simulink model "PWMGenerator"  (R2018a)
settings: Solver=VariableStepAuto  StartTime=0.0  StopTime=10.0  RelTol=1e-3
libraries: hdlsllib x15, simulink x5
settings Model: Creator=prasad.ra  LastModifiedBy=prasad.ra
settings OptimizationCC: BlockReduction=off  ConditionallyExecuteInputs=off  DefaultParameterBehavior=Inlined
settings DebuggingCC: AlgebraicLoopMsg=error
settings HardwareCC: ProdBitPerPointer=32  ProdBitPerSizeT=32  ProdBitPerPtrDiffT=32  ProdLargestAtomicFloat=None  ProdIntDivRoundTo=Undefined  ProdEndianess=Unspecified  ProdWordSize=32  ProdHWDeviceType=ASIC/FPGA->ASIC/FPGA  TargetBitPerPointer=64  TargetBitPerSizeT=64  TargetBitPerPtrDiffT=64  TargetLongLongMode=on  TargetIntDivRoundTo=Zero  TargetEndianess=LittleEndian  TargetWordSize=64  TargetHWDeviceType=Custom Processor->MATLAB Host Computer  ProdEqTarget=off

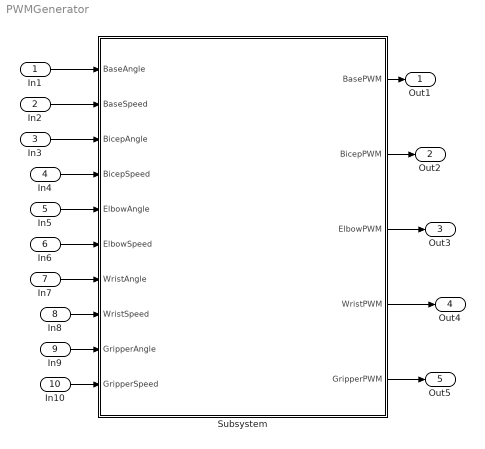
== system PWMGenerator ==
  In1 : Inport
  In2 : Inport  Port=2
  In3 : Inport  Port=3
  In4 : Inport  Port=4
  In5 : Inport  Port=5
  In6 : Inport  Port=6
  In7 : Inport  Port=7
  In8 : Inport  Port=8
  In9 : Inport  Port=9
  In10 : Inport  Port=10
  Subsystem : Subsystem
  Out1 : Outport
  Out2 : Outport  Port=2
  Out3 : Outport  Port=3
  Out4 : Outport  Port=4
  Out5 : Outport  Port=5
  wires:
  In1/1 -> Subsystem/1(BaseAngle)
  In2/1 -> Subsystem/2(BaseSpeed)
  In3/1 -> Subsystem/3(BicepAngle)
  In4/1 -> Subsystem/4(BicepSpeed)
  In7/1 -> Subsystem/7(WristAngle)
  In6/1 -> Subsystem/6(ElbowSpeed)
  In5/1 -> Subsystem/5(ElbowAngle)
  In8/1 -> Subsystem/8(WristSpeed)
  In9/1 -> Subsystem/9(GripperAngle)
  In10/1 -> Subsystem/10(GripperSpeed)
  Subsystem/1(BasePWM) -> Out1/1
  Subsystem/2(BicepPWM) -> Out2/1
  Subsystem/3(ElbowPWM) -> Out3/1
  Subsystem/4(WristPWM) -> Out4/1
  Subsystem/5(GripperPWM) -> Out5/1

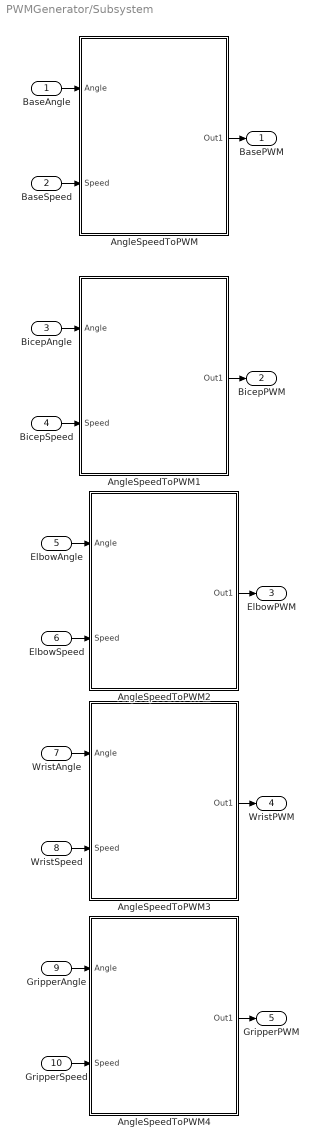
== system PWMGenerator/Subsystem ==
  BaseAngle : Inport
  BaseSpeed : Inport  Port=2
  BicepAngle : Inport  Port=3
  BicepSpeed : Inport  Port=4
  ElbowAngle : Inport  Port=5
  ElbowSpeed : Inport  Port=6
  WristAngle : Inport  Port=7
  WristSpeed : Inport  Port=8
  GripperAngle : Inport  Port=9
  GripperSpeed : Inport  Port=10
  AngleSpeedToPWM : Subsystem
  AngleSpeedToPWM1 : Subsystem
  AngleSpeedToPWM2 : Subsystem
  AngleSpeedToPWM3 : Subsystem
  AngleSpeedToPWM4 : Subsystem
  BasePWM : Outport
  BicepPWM : Outport  Port=2
  ElbowPWM : Outport  Port=3
  WristPWM : Outport  Port=4
  GripperPWM : Outport  Port=5
  wires:
  BicepSpeed/1 -> AngleSpeedToPWM1/2("Speed ")
  AngleSpeedToPWM/1(Out1) -> BasePWM/1
  ElbowSpeed/1 -> AngleSpeedToPWM2/2("Speed ")
  AngleSpeedToPWM2/1(Out1) -> ElbowPWM/1
  BaseAngle/1 -> AngleSpeedToPWM/1(Angle)
  BicepAngle/1 -> AngleSpeedToPWM1/1(Angle)
  AngleSpeedToPWM3/1(Out1) -> WristPWM/1
  AngleSpeedToPWM1/1(Out1) -> BicepPWM/1
  WristSpeed/1 -> AngleSpeedToPWM3/2("Speed ")
  BaseSpeed/1 -> AngleSpeedToPWM/2("Speed ")
  ElbowAngle/1 -> AngleSpeedToPWM2/1(Angle)
  WristAngle/1 -> AngleSpeedToPWM3/1(Angle)
  AngleSpeedToPWM4/1(Out1) -> GripperPWM/1
  GripperAngle/1 -> AngleSpeedToPWM4/1(Angle)
  GripperSpeed/1 -> AngleSpeedToPWM4/2("Speed ")

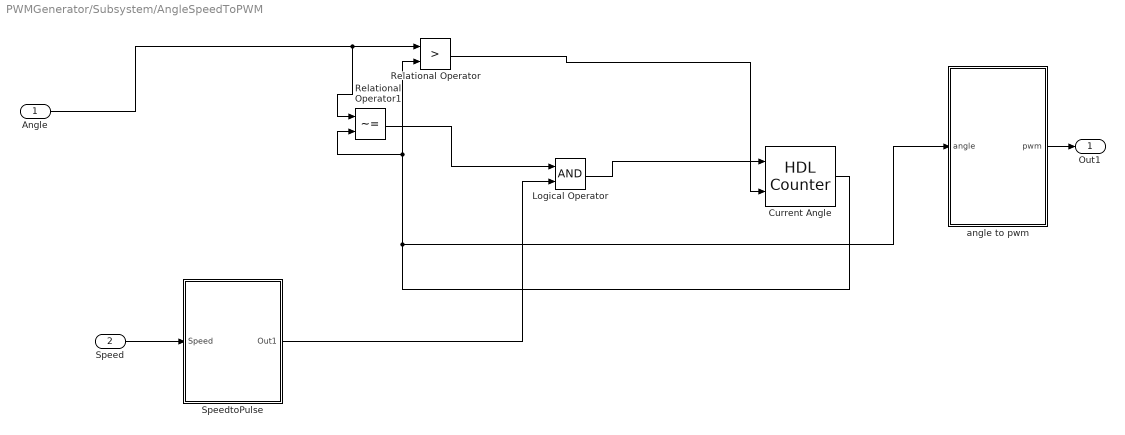
== system PWMGenerator/Subsystem/AngleSpeedToPWM ==
  Angle : Inport
  "Speed " : Inport  Port=2
  "Current Angle " : hdlsllib/Sources/HDL Counter  CountType=Count limited  CountInit=90  CountStep=1  CountMax=180  CountFromType=Specify  CountFrom=0  CountResetPort=off  CountLoadPort=off  CountEnbPort=on  CountDirPort=on  CountDataType=Unsigned  CountWordLen=8  CountFracLen=0  CountSampTime=1
      settings: SourceProductBaseCode=HD
  Logical Operator : Logic  AllPortsSameDT=off  OutDataTypeStr=boolean
  Relational Operator : RelationalOperator  Operator=>  OutDataTypeStr=boolean  RndMeth=Simplest
  Relational Operator1 : RelationalOperator  Operator=~=  OutDataTypeStr=boolean  RndMeth=Simplest
  SpeedtoPulse : Subsystem
  angle to pwm : Subsystem
  Out1 : Outport
  wires:
  Logical Operator/1 -> "Current Angle "/1
  "Current Angle "/1 -> Relational Operator/2, Relational Operator1/2, angle to pwm/1(angle)
  Relational Operator1/1 -> Logical Operator/1
  angle to pwm/1(pwm) -> Out1/1
  SpeedtoPulse/1(Out1) -> Logical Operator/2
  Angle/1 -> Relational Operator/1, Relational Operator1/1
  "Speed "/1 -> SpeedtoPulse/1("Speed ")
  Relational Operator/1 -> "Current Angle "/2

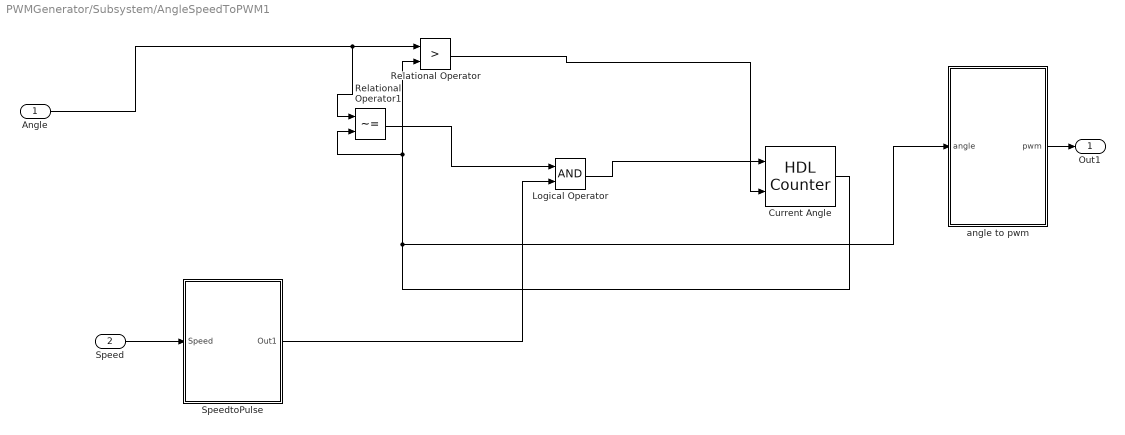
== system PWMGenerator/Subsystem/AngleSpeedToPWM1 ==
  Angle : Inport
  "Speed " : Inport  Port=2
  "Current Angle " : hdlsllib/Sources/HDL Counter  CountType=Count limited  CountInit=90  CountStep=1  CountMax=180  CountFromType=Specify  CountFrom=0  CountResetPort=off  CountLoadPort=off  CountEnbPort=on  CountDirPort=on  CountDataType=Unsigned  CountWordLen=8  CountFracLen=0  CountSampTime=1
      settings: SourceProductBaseCode=HD
  Logical Operator : Logic  AllPortsSameDT=off  OutDataTypeStr=boolean
  Relational Operator : RelationalOperator  Operator=>  OutDataTypeStr=boolean  RndMeth=Simplest
  Relational Operator1 : RelationalOperator  Operator=~=  OutDataTypeStr=boolean  RndMeth=Simplest
  SpeedtoPulse : Subsystem
  angle to pwm : Subsystem
  Out1 : Outport
  wires:
  Logical Operator/1 -> "Current Angle "/1
  "Current Angle "/1 -> Relational Operator/2, Relational Operator1/2, angle to pwm/1(angle)
  Relational Operator1/1 -> Logical Operator/1
  angle to pwm/1(pwm) -> Out1/1
  SpeedtoPulse/1(Out1) -> Logical Operator/2
  Angle/1 -> Relational Operator/1, Relational Operator1/1
  "Speed "/1 -> SpeedtoPulse/1("Speed ")
  Relational Operator/1 -> "Current Angle "/2

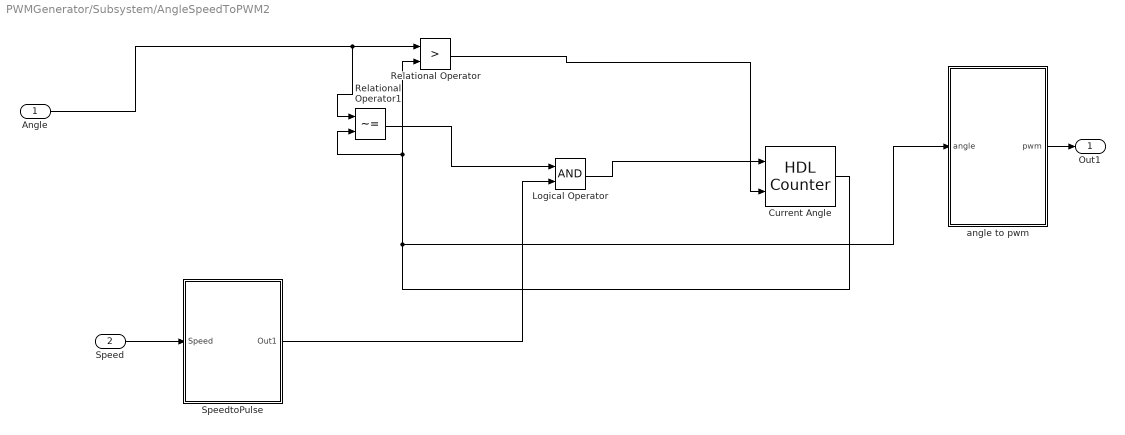
== system PWMGenerator/Subsystem/AngleSpeedToPWM2 ==
  Angle : Inport
  "Speed " : Inport  Port=2
  "Current Angle " : hdlsllib/Sources/HDL Counter  CountType=Count limited  CountInit=90  CountStep=1  CountMax=180  CountFromType=Specify  CountFrom=0  CountResetPort=off  CountLoadPort=off  CountEnbPort=on  CountDirPort=on  CountDataType=Unsigned  CountWordLen=8  CountFracLen=0  CountSampTime=1
      settings: SourceProductBaseCode=HD
  Logical Operator : Logic  AllPortsSameDT=off  OutDataTypeStr=boolean
  Relational Operator : RelationalOperator  Operator=>  OutDataTypeStr=boolean  RndMeth=Simplest
  Relational Operator1 : RelationalOperator  Operator=~=  OutDataTypeStr=boolean  RndMeth=Simplest
  SpeedtoPulse : Subsystem
  angle to pwm : Subsystem
  Out1 : Outport
  wires:
  Logical Operator/1 -> "Current Angle "/1
  "Current Angle "/1 -> Relational Operator/2, Relational Operator1/2, angle to pwm/1(angle)
  Relational Operator1/1 -> Logical Operator/1
  angle to pwm/1(pwm) -> Out1/1
  SpeedtoPulse/1(Out1) -> Logical Operator/2
  Angle/1 -> Relational Operator/1, Relational Operator1/1
  "Speed "/1 -> SpeedtoPulse/1("Speed ")
  Relational Operator/1 -> "Current Angle "/2

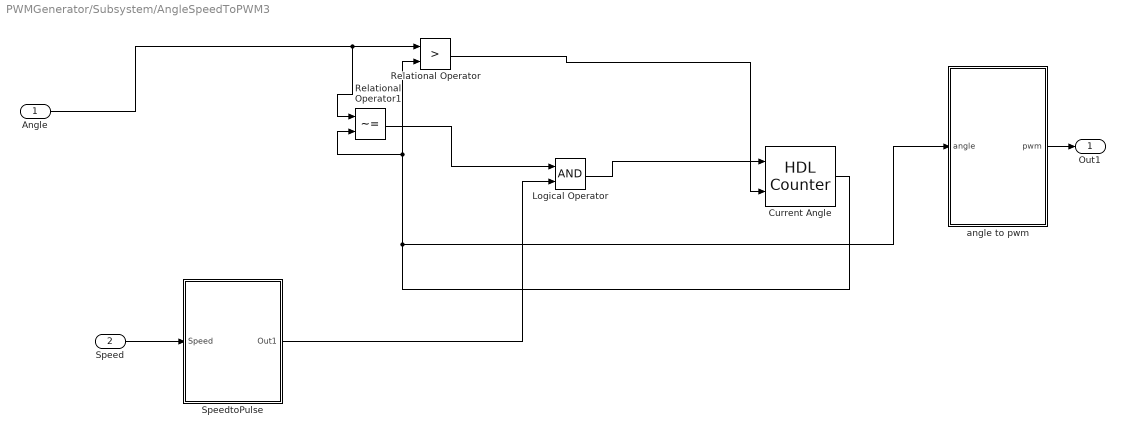
== system PWMGenerator/Subsystem/AngleSpeedToPWM3 ==
  Angle : Inport
  "Speed " : Inport  Port=2
  "Current Angle " : hdlsllib/Sources/HDL Counter  CountType=Count limited  CountInit=90  CountStep=1  CountMax=180  CountFromType=Specify  CountFrom=0  CountResetPort=off  CountLoadPort=off  CountEnbPort=on  CountDirPort=on  CountDataType=Unsigned  CountWordLen=8  CountFracLen=0  CountSampTime=1
      settings: SourceProductBaseCode=HD
  Logical Operator : Logic  AllPortsSameDT=off  OutDataTypeStr=boolean
  Relational Operator : RelationalOperator  Operator=>  OutDataTypeStr=boolean  RndMeth=Simplest
  Relational Operator1 : RelationalOperator  Operator=~=  OutDataTypeStr=boolean  RndMeth=Simplest
  SpeedtoPulse : Subsystem
  angle to pwm : Subsystem
  Out1 : Outport
  wires:
  Logical Operator/1 -> "Current Angle "/1
  "Current Angle "/1 -> Relational Operator/2, Relational Operator1/2, angle to pwm/1(angle)
  Relational Operator1/1 -> Logical Operator/1
  angle to pwm/1(pwm) -> Out1/1
  SpeedtoPulse/1(Out1) -> Logical Operator/2
  Angle/1 -> Relational Operator/1, Relational Operator1/1
  "Speed "/1 -> SpeedtoPulse/1("Speed ")
  Relational Operator/1 -> "Current Angle "/2

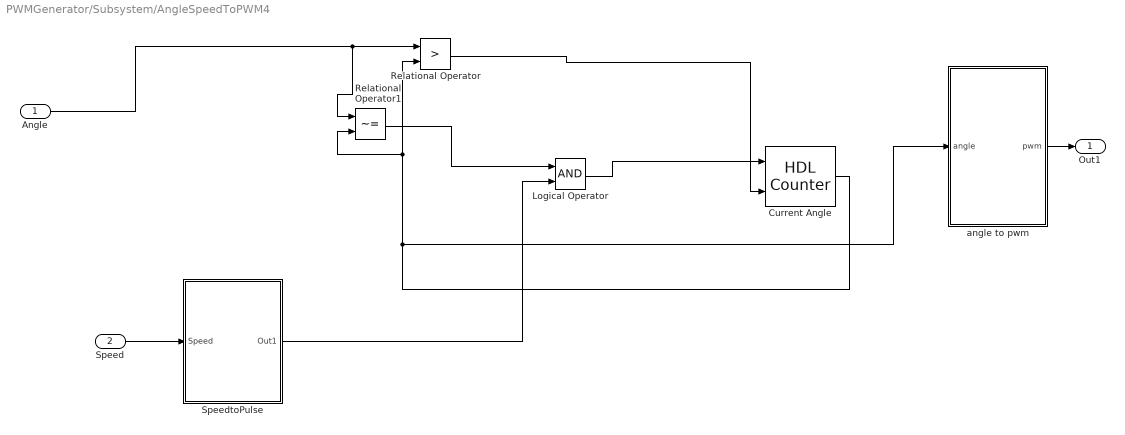
== system PWMGenerator/Subsystem/AngleSpeedToPWM4 ==
  Angle : Inport
  "Speed " : Inport  Port=2
  "Current Angle " : hdlsllib/Sources/HDL Counter  CountType=Count limited  CountInit=90  CountStep=1  CountMax=180  CountFromType=Specify  CountFrom=0  CountResetPort=off  CountLoadPort=off  CountEnbPort=on  CountDirPort=on  CountDataType=Unsigned  CountWordLen=8  CountFracLen=0  CountSampTime=1
      settings: SourceProductBaseCode=HD
  Logical Operator : Logic  AllPortsSameDT=off  OutDataTypeStr=boolean
  Relational Operator : RelationalOperator  Operator=>  OutDataTypeStr=boolean  RndMeth=Simplest
  Relational Operator1 : RelationalOperator  Operator=~=  OutDataTypeStr=boolean  RndMeth=Simplest
  SpeedtoPulse : Subsystem
  angle to pwm : Subsystem
  Out1 : Outport
  wires:
  Logical Operator/1 -> "Current Angle "/1
  "Current Angle "/1 -> Relational Operator/2, Relational Operator1/2, angle to pwm/1(angle)
  Relational Operator1/1 -> Logical Operator/1
  angle to pwm/1(pwm) -> Out1/1
  SpeedtoPulse/1(Out1) -> Logical Operator/2
  Angle/1 -> Relational Operator/1, Relational Operator1/1
  "Speed "/1 -> SpeedtoPulse/1("Speed ")
  Relational Operator/1 -> "Current Angle "/2

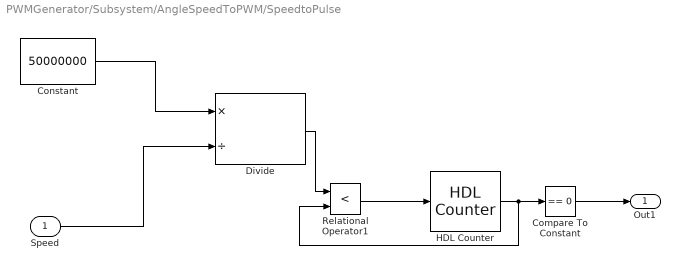
== system PWMGenerator/Subsystem/AngleSpeedToPWM/SpeedtoPulse ==
  "Speed " : Inport  OutDataTypeStr=uint8
  Compare To Constant : simulink/Logic and Bit Operations/Compare To Constant  relop===  const=0  OutDataTypeStr=boolean
  Constant : Constant  Value=50000000  OutDataTypeStr=uint32  SampleTime=1
  Divide : Product  Inputs=*/  SaturateOnIntegerOverflow=on  RndMeth=Zero
  HDL Counter : hdlsllib/Sources/HDL Counter  CountType=Free running  CountInit=0  CountStep=1  CountMax=25  CountFromType=Initial value  CountFrom=0  CountResetPort=on  CountLoadPort=off  CountEnbPort=off  CountDirPort=off  CountDataType=Unsigned  CountWordLen=32  CountFracLen=0  CountSampTime=1
      settings: SourceProductBaseCode=HD
  Relational Operator1 : RelationalOperator  Operator=<  OutDataTypeStr=boolean  RndMeth=Simplest
  Out1 : Outport
  wires:
  "Speed "/1 -> Divide/2
  Compare To Constant/1 -> Out1/1
  Divide/1 -> Relational Operator1/1
  HDL Counter/1 -> Relational Operator1/2, Compare To Constant/1
  Relational Operator1/1 -> HDL Counter/1
  Constant/1 -> Divide/1

== system PWMGenerator/Subsystem/AngleSpeedToPWM/angle to pwm ==
  angle : Inport  OutDataTypeStr=uint8
  Relational Operator : RelationalOperator  Operator=<  OutDataTypeStr=boolean  ZeroCross=off  RndMeth=Simplest
  Subsystem : Subsystem
  pwmCounter : hdlsllib/Sources/HDL Counter  CountType=Count limited  CountInit=0  CountStep=1  CountMax=1000000  CountFromType=Initial value  CountFrom=0  CountResetPort=off  CountLoadPort=off  CountEnbPort=off  CountDirPort=off  CountDataType=Unsigned  CountWordLen=20  CountFracLen=0  CountSampTime=1
      settings: SourceProductBaseCode=HD
  pwm : Outport
  wires:
  Subsystem/1(Out1) -> Relational Operator/2
  Relational Operator/1 -> pwm/1
  pwmCounter/1 -> Relational Operator/1
  angle/1 -> Subsystem/1("angle ")

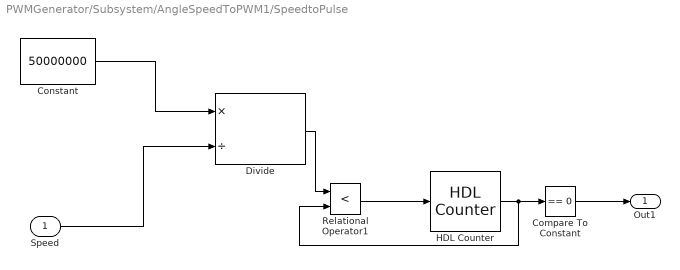
== system PWMGenerator/Subsystem/AngleSpeedToPWM1/SpeedtoPulse ==
  "Speed " : Inport  OutDataTypeStr=uint8
  Compare To Constant : simulink/Logic and Bit Operations/Compare To Constant  relop===  const=0  OutDataTypeStr=boolean
  Constant : Constant  Value=50000000  OutDataTypeStr=uint32  SampleTime=1
  Divide : Product  Inputs=*/  SaturateOnIntegerOverflow=on  RndMeth=Zero
  HDL Counter : hdlsllib/Sources/HDL Counter  CountType=Free running  CountInit=0  CountStep=1  CountMax=25  CountFromType=Initial value  CountFrom=0  CountResetPort=on  CountLoadPort=off  CountEnbPort=off  CountDirPort=off  CountDataType=Unsigned  CountWordLen=32  CountFracLen=0  CountSampTime=1
      settings: SourceProductBaseCode=HD
  Relational Operator1 : RelationalOperator  Operator=<  OutDataTypeStr=boolean  RndMeth=Simplest
  Out1 : Outport
  wires:
  "Speed "/1 -> Divide/2
  Compare To Constant/1 -> Out1/1
  Divide/1 -> Relational Operator1/1
  HDL Counter/1 -> Relational Operator1/2, Compare To Constant/1
  Relational Operator1/1 -> HDL Counter/1
  Constant/1 -> Divide/1

== system PWMGenerator/Subsystem/AngleSpeedToPWM1/angle to pwm ==
  angle : Inport  OutDataTypeStr=uint8
  Relational Operator : RelationalOperator  Operator=<  OutDataTypeStr=boolean  ZeroCross=off  RndMeth=Simplest
  Subsystem : Subsystem
  pwmCounter : hdlsllib/Sources/HDL Counter  CountType=Count limited  CountInit=0  CountStep=1  CountMax=1000000  CountFromType=Initial value  CountFrom=0  CountResetPort=off  CountLoadPort=off  CountEnbPort=off  CountDirPort=off  CountDataType=Unsigned  CountWordLen=20  CountFracLen=0  CountSampTime=1
      settings: SourceProductBaseCode=HD
  pwm : Outport
  wires:
  Subsystem/1(Out1) -> Relational Operator/2
  Relational Operator/1 -> pwm/1
  pwmCounter/1 -> Relational Operator/1
  angle/1 -> Subsystem/1("angle ")

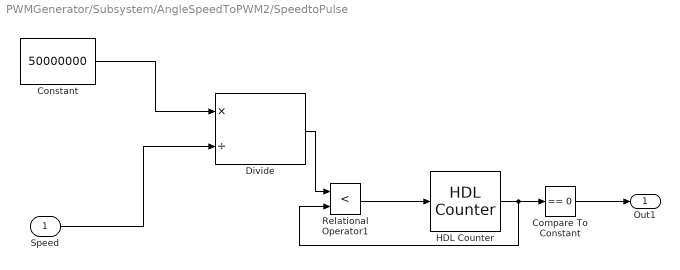
== system PWMGenerator/Subsystem/AngleSpeedToPWM2/SpeedtoPulse ==
  "Speed " : Inport  OutDataTypeStr=uint8
  Compare To Constant : simulink/Logic and Bit Operations/Compare To Constant  relop===  const=0  OutDataTypeStr=boolean
  Constant : Constant  Value=50000000  OutDataTypeStr=uint32  SampleTime=1
  Divide : Product  Inputs=*/  SaturateOnIntegerOverflow=on  RndMeth=Zero
  HDL Counter : hdlsllib/Sources/HDL Counter  CountType=Free running  CountInit=0  CountStep=1  CountMax=25  CountFromType=Initial value  CountFrom=0  CountResetPort=on  CountLoadPort=off  CountEnbPort=off  CountDirPort=off  CountDataType=Unsigned  CountWordLen=32  CountFracLen=0  CountSampTime=1
      settings: SourceProductBaseCode=HD
  Relational Operator1 : RelationalOperator  Operator=<  OutDataTypeStr=boolean  RndMeth=Simplest
  Out1 : Outport
  wires:
  "Speed "/1 -> Divide/2
  Compare To Constant/1 -> Out1/1
  Divide/1 -> Relational Operator1/1
  HDL Counter/1 -> Relational Operator1/2, Compare To Constant/1
  Relational Operator1/1 -> HDL Counter/1
  Constant/1 -> Divide/1

== system PWMGenerator/Subsystem/AngleSpeedToPWM2/angle to pwm ==
  angle : Inport  OutDataTypeStr=uint8
  Relational Operator : RelationalOperator  Operator=<  OutDataTypeStr=boolean  ZeroCross=off  RndMeth=Simplest
  Subsystem : Subsystem
  pwmCounter : hdlsllib/Sources/HDL Counter  CountType=Count limited  CountInit=0  CountStep=1  CountMax=1000000  CountFromType=Initial value  CountFrom=0  CountResetPort=off  CountLoadPort=off  CountEnbPort=off  CountDirPort=off  CountDataType=Unsigned  CountWordLen=20  CountFracLen=0  CountSampTime=1
      settings: SourceProductBaseCode=HD
  pwm : Outport
  wires:
  Subsystem/1(Out1) -> Relational Operator/2
  Relational Operator/1 -> pwm/1
  pwmCounter/1 -> Relational Operator/1
  angle/1 -> Subsystem/1("angle ")

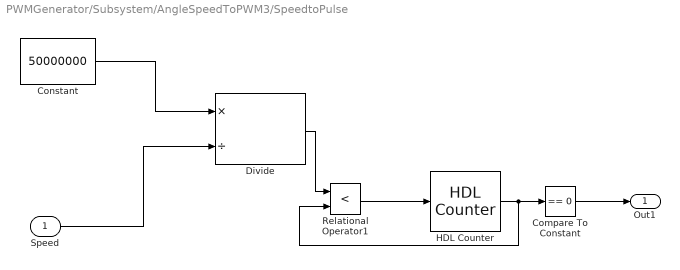
== system PWMGenerator/Subsystem/AngleSpeedToPWM3/SpeedtoPulse ==
  "Speed " : Inport  OutDataTypeStr=uint8
  Compare To Constant : simulink/Logic and Bit Operations/Compare To Constant  relop===  const=0  OutDataTypeStr=boolean
  Constant : Constant  Value=50000000  OutDataTypeStr=uint32  SampleTime=1
  Divide : Product  Inputs=*/  SaturateOnIntegerOverflow=on  RndMeth=Zero
  HDL Counter : hdlsllib/Sources/HDL Counter  CountType=Free running  CountInit=0  CountStep=1  CountMax=25  CountFromType=Initial value  CountFrom=0  CountResetPort=on  CountLoadPort=off  CountEnbPort=off  CountDirPort=off  CountDataType=Unsigned  CountWordLen=32  CountFracLen=0  CountSampTime=1
      settings: SourceProductBaseCode=HD
  Relational Operator1 : RelationalOperator  Operator=<  OutDataTypeStr=boolean  RndMeth=Simplest
  Out1 : Outport
  wires:
  "Speed "/1 -> Divide/2
  Compare To Constant/1 -> Out1/1
  Divide/1 -> Relational Operator1/1
  HDL Counter/1 -> Relational Operator1/2, Compare To Constant/1
  Relational Operator1/1 -> HDL Counter/1
  Constant/1 -> Divide/1

== system PWMGenerator/Subsystem/AngleSpeedToPWM3/angle to pwm ==
  angle : Inport  OutDataTypeStr=uint8
  Relational Operator : RelationalOperator  Operator=<  OutDataTypeStr=boolean  ZeroCross=off  RndMeth=Simplest
  Subsystem : Subsystem
  pwmCounter : hdlsllib/Sources/HDL Counter  CountType=Count limited  CountInit=0  CountStep=1  CountMax=1000000  CountFromType=Initial value  CountFrom=0  CountResetPort=off  CountLoadPort=off  CountEnbPort=off  CountDirPort=off  CountDataType=Unsigned  CountWordLen=20  CountFracLen=0  CountSampTime=1
      settings: SourceProductBaseCode=HD
  pwm : Outport
  wires:
  Subsystem/1(Out1) -> Relational Operator/2
  Relational Operator/1 -> pwm/1
  pwmCounter/1 -> Relational Operator/1
  angle/1 -> Subsystem/1("angle ")

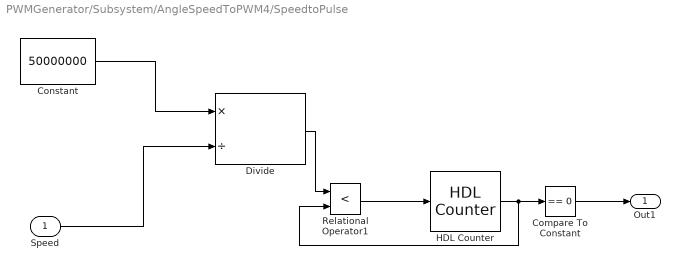
== system PWMGenerator/Subsystem/AngleSpeedToPWM4/SpeedtoPulse ==
  "Speed " : Inport  OutDataTypeStr=uint8
  Compare To Constant : simulink/Logic and Bit Operations/Compare To Constant  relop===  const=0  OutDataTypeStr=boolean
  Constant : Constant  Value=50000000  OutDataTypeStr=uint32  SampleTime=1
  Divide : Product  Inputs=*/  SaturateOnIntegerOverflow=on  RndMeth=Zero
  HDL Counter : hdlsllib/Sources/HDL Counter  CountType=Free running  CountInit=0  CountStep=1  CountMax=25  CountFromType=Initial value  CountFrom=0  CountResetPort=on  CountLoadPort=off  CountEnbPort=off  CountDirPort=off  CountDataType=Unsigned  CountWordLen=32  CountFracLen=0  CountSampTime=1
      settings: SourceProductBaseCode=HD
  Relational Operator1 : RelationalOperator  Operator=<  OutDataTypeStr=boolean  RndMeth=Simplest
  Out1 : Outport
  wires:
  "Speed "/1 -> Divide/2
  Compare To Constant/1 -> Out1/1
  Divide/1 -> Relational Operator1/1
  HDL Counter/1 -> Relational Operator1/2, Compare To Constant/1
  Relational Operator1/1 -> HDL Counter/1
  Constant/1 -> Divide/1

== system PWMGenerator/Subsystem/AngleSpeedToPWM4/angle to pwm ==
  angle : Inport  OutDataTypeStr=uint8
  Relational Operator : RelationalOperator  Operator=<  OutDataTypeStr=boolean  ZeroCross=off  RndMeth=Simplest
  Subsystem : Subsystem
  pwmCounter : hdlsllib/Sources/HDL Counter  CountType=Count limited  CountInit=0  CountStep=1  CountMax=1000000  CountFromType=Initial value  CountFrom=0  CountResetPort=off  CountLoadPort=off  CountEnbPort=off  CountDirPort=off  CountDataType=Unsigned  CountWordLen=20  CountFracLen=0  CountSampTime=1
      settings: SourceProductBaseCode=HD
  pwm : Outport
  wires:
  Subsystem/1(Out1) -> Relational Operator/2
  Relational Operator/1 -> pwm/1
  pwmCounter/1 -> Relational Operator/1
  angle/1 -> Subsystem/1("angle ")

== system PWMGenerator/Subsystem/AngleSpeedToPWM/angle to pwm/Subsystem ==
  "angle " : Inport  OutDataTypeStr=uint8
  Add : Sum
  Constant : Constant  Value=500  OutDataTypeStr=uint16  SampleTime=1
  Constant1 : Constant  Value=30000  OutDataTypeStr=uint32  SampleTime=1
  Product : Product
  Out1 : Outport
  wires:
  Constant/1 -> Product/2
  "angle "/1 -> Product/1
  Product/1 -> Add/1
  Constant1/1 -> Add/2
  Add/1 -> Out1/1

== system PWMGenerator/Subsystem/AngleSpeedToPWM1/angle to pwm/Subsystem ==
  "angle " : Inport  OutDataTypeStr=uint8
  Add : Sum
  Constant : Constant  Value=500  OutDataTypeStr=uint16  SampleTime=1
  Constant1 : Constant  Value=30000  OutDataTypeStr=uint32  SampleTime=1
  Product : Product
  Out1 : Outport
  wires:
  Constant/1 -> Product/2
  "angle "/1 -> Product/1
  Product/1 -> Add/1
  Constant1/1 -> Add/2
  Add/1 -> Out1/1

== system PWMGenerator/Subsystem/AngleSpeedToPWM2/angle to pwm/Subsystem ==
  "angle " : Inport  OutDataTypeStr=uint8
  Add : Sum
  Constant : Constant  Value=500  OutDataTypeStr=uint16  SampleTime=1
  Constant1 : Constant  Value=30000  OutDataTypeStr=uint32  SampleTime=1
  Product : Product
  Out1 : Outport
  wires:
  Constant/1 -> Product/2
  "angle "/1 -> Product/1
  Product/1 -> Add/1
  Constant1/1 -> Add/2
  Add/1 -> Out1/1

== system PWMGenerator/Subsystem/AngleSpeedToPWM3/angle to pwm/Subsystem ==
  "angle " : Inport  OutDataTypeStr=uint8
  Add : Sum
  Constant : Constant  Value=500  OutDataTypeStr=uint16  SampleTime=1
  Constant1 : Constant  Value=30000  OutDataTypeStr=uint32  SampleTime=1
  Product : Product
  Out1 : Outport
  wires:
  Constant/1 -> Product/2
  "angle "/1 -> Product/1
  Product/1 -> Add/1
  Constant1/1 -> Add/2
  Add/1 -> Out1/1

== system PWMGenerator/Subsystem/AngleSpeedToPWM4/angle to pwm/Subsystem ==
  "angle " : Inport  OutDataTypeStr=uint8
  Add : Sum
  Constant : Constant  Value=500  OutDataTypeStr=uint16  SampleTime=1
  Constant1 : Constant  Value=30000  OutDataTypeStr=uint32  SampleTime=1
  Product : Product
  Out1 : Outport
  wires:
  Constant/1 -> Product/2
  "angle "/1 -> Product/1
  Product/1 -> Add/1
  Constant1/1 -> Add/2
  Add/1 -> Out1/1
